simulink model "rtwdemo_atomic"  (Simulink 7.6)
settings: Solver=FixedStepDiscrete  StartTime=0.0  StopTime=10.0  FixedStep=1  RelTol=1e-3
undefined symbols (not defined in the file or in its folder): DiscIntNeverNeededParam
libraries: rtwdemowidgets x2
Description:
  | Preserving Subsystem Boundaries in Generated Code
settings Model: Creator=The MathWorks Inc.  ExtModeAutoUpdateStatusClock=off
settings MATStruct: SampleTime=1  Offset=0  Priority=[20.0]
settings DataIOCC: SaveOutput=off  SaveTime=off  SignalLoggingName=sigsOut
settings OptimizationCC: InlineParams=on  InlineInvariantSignals=on  StateBitsets=on  DataBitsets=on  UseTempVars=on  EfficientFloat2IntCast=on  EfficientMapNaN2IntZero=off
settings DebuggingCC: CheckExecutionContextPreStartOutputMsg=on  CheckExecutionContextRuntimeOutputMsg=on  SolverPrmCheckMsg=none  StrictBusMsg=ErrorOnBusTreatedAsVector
settings HardwareCC: ProdIntDivRoundTo=Zero  ProdEndianess=LittleEndian  ProdHWDeviceType=Generic->32-bit Embedded Processor  TargetHWDeviceType=Generic->32-bit Embedded Processor
settings RTWCC: TLCOptions=-p0 -aWarnNonSaturatedBlocks=0  GenerateReport=on  RTWVerbose=off  ProcessScript=grt_make_rtw_hook  LaunchReport=on
settings CodeAppCC: ForceParamTrailComments=on
settings GRTTargetCC: TargetFcnLib=ansi_tfl_tmw.mat

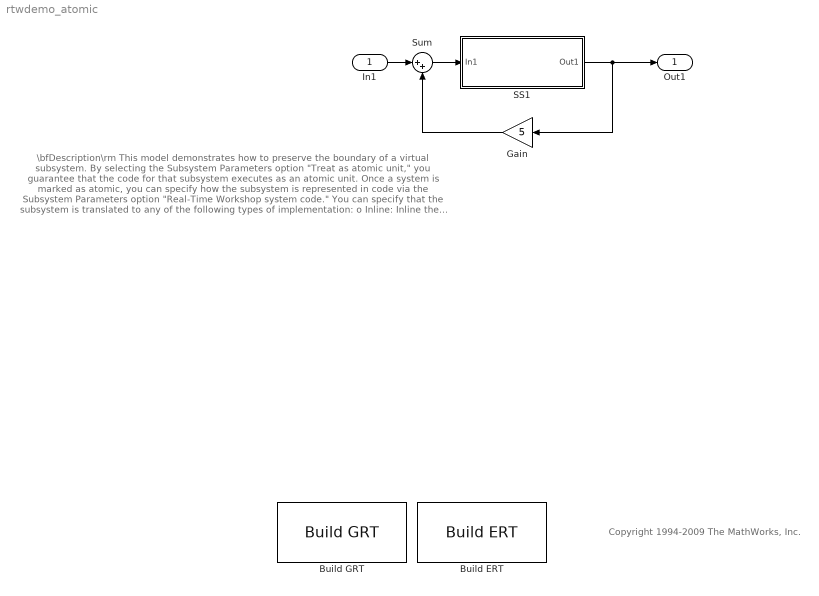
== system rtwdemo_atomic ==
  note: \bfDescription\rm
      | This model demonstrates how to preserve the boundary of a virtual subsystem.  By selecting the
      | Subsystem Parameters option "Treat as atomic unit," you guarantee that the code for that subsystem
      | executes as an atomic unit.  Once a system is marked as atomic, you can specify how the subsystem
      | is represented in code via the Subsystem Parameters option "Real-Time Workshop system code."
      | You can specify that the subsystem is translated to any of the following types of implementation:
      |
      | o  Inline:  Inline the subsystem code at the call sites
      | o  Function:  A void/void function with I/O and internal data in global data structure
      | o  Reusable Function:  A re-entrant function with data passed in as part of function arguments
      | o  Auto:  Let Real-Time Workshop optimize the implementation based on context
      |
      | \bfInstructions\rm
      | 1. Generate code by double-clicking the blue buttons below.  An HTML report is displayed automatically.
      | 2. Inspect rtwdemo\_atomic.c:  SS1 is configured as a "Reusable function" with function name "myfun".
      |
      | \bfNote\rm
      | Simulink and Real-Time Workshop can avoid "artificial" algebraic loops when the subsystem
      | is made atomic via the subsystem option "Minimize algebraic loop occurrences."  See the
      | Simulink documentation for information on minimizing occurrences of algebraic loops.
  note: Copyright 1994-2009 The MathWorks, Inc.
  In1 : Inport  OutDataTypeStr=double  PortDimensions=1  SampleTime=1
  Build ERT : rtwdemowidgets/Build ERT  SystemSampleTime=-1  attrib_overrides={}
  Build GRT : rtwdemowidgets/Build GRT  SystemSampleTime=-1  attrib_overrides={}
  Gain : Gain  Gain=5  SaturateOnIntegerOverflow=on  OutDataTypeStr=Inherit: Same as input  ParamDataTypeStr=Inherit: Same as input
  SS1 : Subsystem  TreatAsAtomicUnit=on  RTWFcnName=myfun  RTWFileName=myfile
      settings: RTWFcnNameOpts=User specified
  Sum : Sum  Inputs=|++
  Out1 : Outport
  wires:
  Sum/1 -> SS1/1(In1)
  In1/1 -> Sum/1
  SS1/1(Out1) -> Out1/1, Gain/1
  Gain/1 -> Sum/2

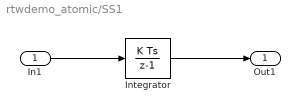
== system rtwdemo_atomic/SS1 ==
  In1 : Inport
  Integrator : DiscreteIntegrator  InitialConditionMode=State only (most efficient)  ICPrevOutput=DiscIntNeverNeededParam  ICPrevScaledInput=DiscIntNeverNeededParam
  Out1 : Outport
  wires:
  In1/1 -> Integrator/1
  Integrator/1 -> Out1/1
